simulink model "PILnewH2019"  (R2021a)
settings: Solver=FixedStepAuto  StartTime=0.0  StopTime=41.24  FixedStep=0.001  RelTol=1e-3  EnableMultiTasking=on
values from neighbouring files (symbols this model uses):
  den_lpf_d = den_lpf20    [Mainframe_init.m]    (also in load_autopilot.m)
  Emulated_FCC_IO_Delay = 7    [Mainframe_init.m]
  Enable_Gyros = 0    [Mainframe_init.m]
  Enable_INS = 0    [Mainframe_init.m]
  num_lpf_d = num_lpf20    [Mainframe_init.m]    (also in load_autopilot.m)
undefined symbols (not defined in the file or in its folder): act_dmp, act_omega, Actuator, Aerodynamics, aMode, Autopilot, AUX, c_b_WGS, c_be, c_flat, c_grav, c_h_geop0, c_h_geope, c_pa0, c_pe, c_r0, c_rot, c_rsma, c_Tmp0, d_siB_0, d_siB_max, d_siB_min, dd_siB_max, dd_siB_min, dev, DiscIntNeverNeededParam, e_pa, e_Tmp, Earth, fin_maxrate, flag_I_act_switch, flag_I_aero_switch, flag_I_flat, flag_I_gravity_switch, flag_I_rot, hcr, HIL_Data, JMMM_0, JMMM_e, JSPB_e, lat_0, lon_0, Mass_Props, mB_0, mM_0, mM_e, National_Instruments, pBII_0, PCIe, pMPB, pNPB, propellant_kg, prp_FBPB, prp_mdot, prp_T, pSPB, pwm_output1, qEG_0, qIB_0, qIE_0 ... (+29)
libraries: simulink x31, simulink_extras x24, aerolibcommonsys x4, px4lib x2, custom_blocks x1, pil_lib x1, aerolibtransform2 x1, sldrtlib x1, aerolibnav x1
(part 10 of 15)

== system PILnewH2019/Non-linear Flight Dynamic Model/Subsystem1/GRM_Airframe/stream_flow/calc_stream_flow/velocity_vector_transformation ==
  wIEE : Inport
  TIE : Inport  Port=2
  vBII : Inport  Port=3
  pBII : Inport  Port=4
  Add : Sum  Inputs=+-
  Product : Product  Multiplication=Matrix(*)
  cross_product : Subsystem
      mask help: cross product r3 = r1 x r2
      mask Help:
      | Name:
      | 
      |     cross_product
      | 
      | Description:
      | 
      |     This block implements the cross product r3 = r1 x r2.
      | 
      | Inputs  [size] [data type] [unit]:
      | 
      |     vector 1  [3] [double] [-]
      |     vector 2  [3] [double] [-]
      | 
      | Outputs  [size] [data type] [unit]:
      | 
      |     resulting vector  [3] [double] [-]
      mask Display: disp(' r3 = r1 x r2')
  vBEI : Outport  VectorParamsAs1DForOutWhenUnconnected=off
  wires:
  TIE/1 -> Product/1
  wIEE/1 -> Product/2
  Product/1 -> cross_product/1(r1)  "wIEI"
  pBII/1 -> cross_product/2(r2)
  cross_product/1(r1_x_r2) -> Add/2  "de_vBEI"
  vBII/1 -> Add/1
  Add/1 -> vBEI/1  "vBEI"

== system PILnewH2019/Non-linear Flight Dynamic Model/Subsystem1/GRM_Airframe/weight_and_balance/moi/JMMM_linear_interpolation ==
  mM : Inport
  Constant16 : Constant  Value=JMMM_0
  Constant17 : Constant  Value=JMMM_e
  Constant18 : Constant  Value=mM_0
  Constant19 : Constant  Value=mM_e
  Constant20 : Constant  Value=mM_0
  Constant21 : Constant  Value=JMMM_0
  Divide : Product  Inputs=**/
  Subtract : Sum  Inputs=+-
  Subtract4 : Sum  Inputs=+-
  Subtract5 : Sum  Inputs=+-
  Subtract6 : Sum
  JMMM : Outport  VectorParamsAs1DForOutWhenUnconnected=off
  wires:
  mM/1 -> Subtract5/1
  Subtract5/1 -> Divide/1
  Constant20/1 -> Subtract5/2
  Constant19/1 -> Subtract4/1
  Constant18/1 -> Subtract4/2
  Constant17/1 -> Subtract/1
  Constant16/1 -> Subtract/2
  Subtract/1 -> Divide/2
  Subtract4/1 -> Divide/3
  Subtract6/1 -> JMMM/1  "JMMM"
  Constant21/1 -> Subtract6/1
  Divide/1 -> Subtract6/2

== system PILnewH2019/Non-linear Flight Dynamic Model/Subsystem1/GRM_Airframe/weight_and_balance/moi/moi_coordinate_transformation ==
  JMMM : Inport
  3_rot_mat : Subsystem  mask(Rotation um 1, 2 oder 3 Achsen){rot_1=Rotation um z-Achse, rot_2=Rotation um y-Achse, rot_3=Rotation um x-Achse}
      mask prompts: rot_1 "1. Rotation"; rot_2 "2. Rotation"; rot_3 "3. Rotation"
      mask help:
      | Dieser Block liefert die Rotationsmatrix T12 für den Fall zurück, dass sich das Ziel-Koordinatensystem (1) durch Drehungen um 1, 2 oder 3 Achsen gegenüber dem Ausgangskoordinatensystem (2) beschreiben lässt (passive Drehung).
      |
      | Die Anzahl der Rotation sowie die Reihenfolge ist frei einstellbar.
      |
      | Die Rotationswinkel haben die Einheit [rad].
      mask TypeOptions rot_1: Rotation um x-Achse | Rotation um y-Achse | Rotation um z-Achse
      mask TypeOptions rot_2: Rotation um x-Achse | Rotation um y-Achse | Rotation um z-Achse
      mask TypeOptions rot_3: Rotation um x-Achse | Rotation um y-Achse | Rotation um z-Achse
  Math Function : Math  Operator=transpose  SignedPower=on  SaturateOnIntegerOverflow=on
  Matrix Multiply : Product  Multiplication=Matrix(*)
  Matrix Multiply1 : Product  Multiplication=Matrix(*)
  Thrust_rot_z : Constant  Value=unc_prp_z
  thrust_rot_x : Constant  Value=unc_prp_x
  thrust_rot_y : Constant  Value=unc_prp_y
  JMMB : Outport  VectorParamsAs1DForOutWhenUnconnected=off
  wires:
  Math Function/1 -> Matrix Multiply1/2
  Matrix Multiply/1 -> Matrix Multiply1/1
  JMMM/1 -> Matrix Multiply/2
  3_rot_mat/1(T12) -> Math Function/1, Matrix Multiply/1
  Matrix Multiply1/1 -> JMMB/1  "JMMB"
  thrust_rot_y/1 -> 3_rot_mat/2(wi2)
  thrust_rot_x/1 -> 3_rot_mat/3(wi3)
  Thrust_rot_z/1 -> 3_rot_mat/1(wi1)

== system PILnewH2019/Non-linear Flight Dynamic Model/Subsystem1/GRM_Airframe/weight_and_balance/moi/moi_uncertainty ==
  JBBB_c : Inport
  Add7 : Sum
  Constant16 : Constant  Value=[unc_moi_Jxx,0,0;0,unc_moi_Jyy,0;0,0,unc_moi_Jzz]
  JBBB : Outport  VectorParamsAs1DForOutWhenUnconnected=off
  wires:
  Add7/1 -> JBBB/1  "JBBB"
  JBBB_c/1 -> Add7/1
  Constant16/1 -> Add7/2

== system PILnewH2019/Non-linear Flight Dynamic Model/Subsystem1/GRM_Airframe/weight_and_balance/moi/steiners_theorem_missile ==
  pBPB : Inport
  Constant : Constant  Value=mB_0
  Constant17 : Constant  Value=pSPB
  Product : Product
  Subtract : Sum  Inputs=+-
  create_deviation_matrix : Subsystem
  J_deviation : Outport  VectorParamsAs1DForOutWhenUnconnected=off
  wires:
  pBPB/1 -> Subtract/1
  Product/1 -> J_deviation/1
  create_deviation_matrix/1(T_deviation) -> Product/2
  Constant17/1 -> Subtract/2
  Subtract/1 -> create_deviation_matrix/1(pBXB)  "pB0B"
  Constant/1 -> Product/1

== system PILnewH2019/Non-linear Flight Dynamic Model/Subsystem1/GRM_Airframe/weight_and_balance/moi/steiners_theorem_motor ==
  pBPB : Inport
  mM : Inport  Port=2
  Constant16 : Constant  Value=pMPB
  Product : Product
  Subtract4 : Sum  Inputs=+-
  create_deviation_matrix1 : Subsystem
  JM_deviation : Outport  VectorParamsAs1DForOutWhenUnconnected=off
  wires:
  Product/1 -> JM_deviation/1
  pBPB/1 -> Subtract4/1
  create_deviation_matrix1/1(T_deviation) -> Product/1
  Constant16/1 -> Subtract4/2
  Subtract4/1 -> create_deviation_matrix1/1(pBXB)  "pBMB"
  mM/1 -> Product/2

== system PILnewH2019/Flight Control Computer/FCC - Real or Emulated/Emulated FCC/PixBlock3/Emulated Pixhawk/Autopilot/Calculate U ==
  INS Data : Inport
  Add : Sum  Inputs=+++
  Bus Selector1 : BusSelector  OutputSignals=u,v,w
  Square : Math  Operator=square  SaturateOnIntegerOverflow=on
  Square Root : Sqrt  SaturateOnIntegerOverflow=on
  Square1 : Math  Operator=square  SaturateOnIntegerOverflow=on
  Square2 : Math  Operator=square  SaturateOnIntegerOverflow=on
  U : Outport
  wires:
  Square/1 -> Add/1
  Square2/1 -> Add/3
  Square Root/1 -> U/1
  Add/1 -> Square Root/1
  Square1/1 -> Add/2
  Bus Selector1/2 -> Square1/1  "<v>"
  Bus Selector1/3 -> Square2/1  "<w>"
  Bus Selector1/1 -> Square/1  "<u>"
  INS Data/1 -> Bus Selector1/1

== system PILnewH2019/Flight Control Computer/FCC - Real or Emulated/Emulated FCC/PixBlock3/Emulated Pixhawk/Autopilot/Phi_Control ==
  phi_cmd_rad : Inport
  phi_rad : Inport  Port=2
  p_rps : Inport  Port=3
  Reset Integrators : Inport  Port=4
  V_mps : Inport  Port=5
  h_m : Inport  Port=6
  Bus Selector : BusSelector  OutputSignals=Kp_p,Ki_phi,Kp_phi,Kp_r,Ki_ay,Kp_ay
  Constant : Constant  Value=0  OutDataTypeStr=single
  Discrete-Time Integrator : DiscreteIntegrator  ExternalReset=level  InitialConditionSource=external  SampleTime=-1  OutDataTypeStr=single  ICPrevOutput=DiscIntNeverNeededParam  ICPrevScaledInput=DiscIntNeverNeededParam
  Gain_Lookup : Subsystem
  Product1 : Product
  Product2 : Product
  Product3 : Product
  Sum3 : Sum  Inputs=|+-
  Sum4 : Sum  Inputs=++|
  Sum5 : Sum  Inputs=|+-
  dela_cmd_rad : Outport
  wires:
  phi_cmd_rad/1 -> Sum3/1
  Reset Integrators/1 -> Discrete-Time Integrator/2
  p_rps/1 -> Sum5/2
  phi_rad/1 -> Sum3/2
  Product2/1 -> Sum4/1
  Sum3/1 -> Product3/2, Product2/2
  Constant/1 -> Discrete-Time Integrator/3
  Sum5/1 -> Product1/2
  [Ki_phi] -> Product3/1
  Product1/1 -> dela_cmd_rad/1
  [Kp_p] -> Product1/1
  [Kp_phi] -> Product2/1
  Discrete-Time Integrator/1 -> Sum4/2  "phi_int"
  Sum4/1 -> Sum5/1
  Product3/1 -> Discrete-Time Integrator/1
  h_m/1 -> Gain_Lookup/2(h_m)
  Bus Selector/6 -> [Kp_ay]  "<Kp_ay>"
  Bus Selector/5 -> [Ki_ay]  "<Ki_ay>"
  Bus Selector/2 -> [Ki_phi]  "<Ki_phi>"
  Bus Selector/1 -> [Kp_p]  "<Kp_p>"
  V_mps/1 -> Gain_Lookup/1(V_mps)
  Bus Selector/4 -> [Kp_r]  "<Kp_r>"
  Gain_Lookup/1(Gains) -> Bus Selector/1
  Bus Selector/3 -> [Kp_phi]  "<Kp_phi>"

== system PILnewH2019/Flight Control Computer/FCC - Real or Emulated/Emulated FCC/PixBlock3/Emulated Pixhawk/Convert to Bus/100Hz Reset ==
  Heartbeat : Inport
  Delay : Delay  DelayLength=1
  GreaterThan : RelationalOperator  Operator=<  OutDataTypeStr=boolean  RndMeth=Simplest
  RST : Outport
  wires:
  GreaterThan/1 -> RST/1
  Delay/1 -> GreaterThan/2
  Heartbeat/1 -> Delay/1, GreaterThan/1

== system PILnewH2019/Flight Control Computer/FCC - Real or Emulated/Emulated FCC/PixBlock3/Emulated Pixhawk/Fin Allocation/control_allocation ==
  fin_cmd : Inport
  Constant7 : Constant  Value=HIL_Data.FDM.Tr4r3  OutDataTypeStr=single
  Product : Product  Multiplication=Matrix(*)
  siB_cmd : Outport  VectorParamsAs1DForOutWhenUnconnected=off
  wires:
  Constant7/1 -> Product/1
  fin_cmd/1 -> Product/2
  Product/1 -> siB_cmd/1  "siB_cmd"

== system PILnewH2019/Flight Control Computer/FCC - Real or Emulated/Emulated FCC/PixBlock3/Emulated Pixhawk/Inertial Navigation System/INS (INCOMPLETE) ==
  IMU Data : Inport
  Bus Creator2 : BusCreator  Inputs=12
  One{,1..11} (12 alike) : Constant  Value=-1  OutDataTypeStr=Inherit: Inherit via back propagation
  Terminator : Terminator
  INS Data : Outport
  wires:
  One11/1 -> Bus Creator2/12  "psi"
  One10/1 -> Bus Creator2/11  "theta"
  One9/1 -> Bus Creator2/10  "phi"
  One8/1 -> Bus Creator2/9  "r"
  One7/1 -> Bus Creator2/8  "q"
  One2/1 -> Bus Creator2/3  "w"
  One6/1 -> Bus Creator2/7  "p"
  One4/1 -> Bus Creator2/5  "y"
  One1/1 -> Bus Creator2/2  "v"
  One5/1 -> Bus Creator2/6  "z"
  One/1 -> Bus Creator2/1  "u"
  One3/1 -> Bus Creator2/4  "x"
  IMU Data/1 -> Terminator/1
  Bus Creator2/1 -> INS Data/1

== system PILnewH2019/Flight Control Computer/FCC - Real or Emulated/Emulated FCC/PixBlock3/Emulated Pixhawk/Servo Commands/100Hz Progress ==
  Delay : Delay  DelayLength=1
  GreaterThan : RelationalOperator  Operator=>  OutDataTypeStr=boolean  RndMeth=Simplest
  RST : Outport
  wires:
  GreaterThan/1 -> RST/1
  Delay/1 -> GreaterThan/2
  [Heartbeat] -> Delay/1, GreaterThan/1

== system PILnewH2019/Flight Control Computer/FCC - Real or Emulated/Real FCC/PixBlock2/Emulated Pixhawk/Autopilot/Calculate U ==
  INS Data : Inport
  Add : Sum  Inputs=+++
  Bus Selector1 : BusSelector  OutputSignals=u,v,w
  Square : Math  Operator=square  SaturateOnIntegerOverflow=on
  Square Root : Sqrt  SaturateOnIntegerOverflow=on
  Square1 : Math  Operator=square  SaturateOnIntegerOverflow=on
  Square2 : Math  Operator=square  SaturateOnIntegerOverflow=on
  U : Outport
  wires:
  Square/1 -> Add/1
  Square2/1 -> Add/3
  Square Root/1 -> U/1
  Add/1 -> Square Root/1
  Square1/1 -> Add/2
  Bus Selector1/2 -> Square1/1  "<v>"
  Bus Selector1/3 -> Square2/1  "<w>"
  Bus Selector1/1 -> Square/1  "<u>"
  INS Data/1 -> Bus Selector1/1

== system PILnewH2019/Flight Control Computer/FCC - Real or Emulated/Real FCC/PixBlock2/Emulated Pixhawk/Autopilot/Phi_Control ==
  phi_cmd_rad : Inport
  phi_rad : Inport  Port=2
  p_rps : Inport  Port=3
  Reset Integrators : Inport  Port=4
  V_mps : Inport  Port=5
  h_m : Inport  Port=6
  Bus Selector : BusSelector  OutputSignals=Kp_p,Ki_phi,Kp_phi,Kp_r,Ki_ay,Kp_ay
  Constant : Constant  Value=0  OutDataTypeStr=single
  Discrete-Time Integrator : DiscreteIntegrator  ExternalReset=level  InitialConditionSource=external  SampleTime=-1  OutDataTypeStr=single  ICPrevOutput=DiscIntNeverNeededParam  ICPrevScaledInput=DiscIntNeverNeededParam
  Gain_Lookup : Subsystem
  Product1 : Product
  Product2 : Product
  Product3 : Product
  Sum3 : Sum  Inputs=|+-
  Sum4 : Sum  Inputs=++|
  Sum5 : Sum  Inputs=|+-
  dela_cmd_rad : Outport
  wires:
  phi_cmd_rad/1 -> Sum3/1
  Reset Integrators/1 -> Discrete-Time Integrator/2
  p_rps/1 -> Sum5/2
  phi_rad/1 -> Sum3/2
  Product2/1 -> Sum4/1
  Sum3/1 -> Product3/2, Product2/2
  Constant/1 -> Discrete-Time Integrator/3
  Sum5/1 -> Product1/2
  [Ki_phi] -> Product3/1
  Product1/1 -> dela_cmd_rad/1
  [Kp_p] -> Product1/1
  [Kp_phi] -> Product2/1
  Discrete-Time Integrator/1 -> Sum4/2  "phi_int"
  Sum4/1 -> Sum5/1
  Product3/1 -> Discrete-Time Integrator/1
  h_m/1 -> Gain_Lookup/2(h_m)
  Bus Selector/6 -> [Kp_ay]  "<Kp_ay>"
  Bus Selector/5 -> [Ki_ay]  "<Ki_ay>"
  Bus Selector/2 -> [Ki_phi]  "<Ki_phi>"
  Bus Selector/1 -> [Kp_p]  "<Kp_p>"
  V_mps/1 -> Gain_Lookup/1(V_mps)
  Bus Selector/4 -> [Kp_r]  "<Kp_r>"
  Gain_Lookup/1(Gains) -> Bus Selector/1
  Bus Selector/3 -> [Kp_phi]  "<Kp_phi>"

== system PILnewH2019/Flight Control Computer/FCC - Real or Emulated/Real FCC/PixBlock2/Emulated Pixhawk/Convert to Bus/100Hz Reset ==
  Heartbeat : Inport
  Delay : Delay  DelayLength=1
  GreaterThan : RelationalOperator  Operator=<  OutDataTypeStr=boolean  RndMeth=Simplest
  RST : Outport
  wires:
  GreaterThan/1 -> RST/1
  Delay/1 -> GreaterThan/2
  Heartbeat/1 -> Delay/1, GreaterThan/1

== system PILnewH2019/Flight Control Computer/FCC - Real or Emulated/Real FCC/PixBlock2/Emulated Pixhawk/Fin Allocation/control_allocation ==
  fin_cmd : Inport
  Constant7 : Constant  Value=HIL_Data.FDM.Tr4r3  OutDataTypeStr=single
  Product : Product  Multiplication=Matrix(*)
  siB_cmd : Outport  VectorParamsAs1DForOutWhenUnconnected=off
  wires:
  Constant7/1 -> Product/1
  fin_cmd/1 -> Product/2
  Product/1 -> siB_cmd/1  "siB_cmd"

== system PILnewH2019/Flight Control Computer/FCC - Real or Emulated/Real FCC/PixBlock2/Emulated Pixhawk/Inertial Navigation System/INS (INCOMPLETE) ==
  IMU Data : Inport
  Bus Creator2 : BusCreator  Inputs=12
  One{,1..11} (12 alike) : Constant  Value=-1  OutDataTypeStr=Inherit: Inherit via back propagation
  Terminator : Terminator
  INS Data : Outport
  wires:
  One11/1 -> Bus Creator2/12  "psi"
  One10/1 -> Bus Creator2/11  "theta"
  One9/1 -> Bus Creator2/10  "phi"
  One8/1 -> Bus Creator2/9  "r"
  One7/1 -> Bus Creator2/8  "q"
  One2/1 -> Bus Creator2/3  "w"
  One6/1 -> Bus Creator2/7  "p"
  One4/1 -> Bus Creator2/5  "y"
  One1/1 -> Bus Creator2/2  "v"
  One5/1 -> Bus Creator2/6  "z"
  One/1 -> Bus Creator2/1  "u"
  One3/1 -> Bus Creator2/4  "x"
  IMU Data/1 -> Terminator/1
  Bus Creator2/1 -> INS Data/1

== system PILnewH2019/Flight Control Computer/FCC - Real or Emulated/Real FCC/PixBlock2/Emulated Pixhawk/Servo Commands/100Hz Progress ==
  Delay : Delay  DelayLength=1
  GreaterThan : RelationalOperator  Operator=>  OutDataTypeStr=boolean  RndMeth=Simplest
  RST : Outport
  wires:
  GreaterThan/1 -> RST/1
  Delay/1 -> GreaterThan/2
  [Heartbeat] -> Delay/1, GreaterThan/1

== system PILnewH2019/Non-linear Flight Dynamic Model/Extract States/Assemble_States_Bus1/Three-axis Inertial Measurement Unit3/Three-axis Accelerometer/Dynamics/No Dynamics ==
  In1 : Inport
  Out1 : Outport  VectorParamsAs1DForOutWhenUnconnected=off
  wires:
  In1/1 -> Out1/1

== system PILnewH2019/Non-linear Flight Dynamic Model/Extract States/Assemble_States_Bus1/Three-axis Inertial Measurement Unit3/Three-axis Accelerometer/Dynamics/Second-order Dynamics ==
  In : Inport
  2*zeta * wn : Gain  Gain=2.0*zn*wn  SaturateOnIntegerOverflow=on  OutDataTypeStr=Inherit: Same as input  ParamDataTypeStr=Inherit: Same as input
  "Integrator, Second-Order Limited" : SecondOrderIntegrator  ICX=0  UpperLimitX=fin_max  LowerLimitX=fin_min  ICDXDT=0  UpperLimitDXDT=fin_maxrate  LowerLimitDXDT=-fin_maxrate
  Sum2 : Sum  Inputs=|+-  InputSameDT=on  SaturateOnIntegerOverflow=on  OutDataTypeStr=Inherit: Same as first input
  Sum3 : Sum  Inputs=|+-  InputSameDT=on  SaturateOnIntegerOverflow=on  OutDataTypeStr=Inherit: Same as first input
  wn^2 : Gain  Gain=wn*wn  SaturateOnIntegerOverflow=on  OutDataTypeStr=Inherit: Same as input  ParamDataTypeStr=Inherit: Same as input
  Out : Outport  VectorParamsAs1DForOutWhenUnconnected=off
  wires:
  "Integrator, Second-Order Limited"/2 -> 2*zeta * wn/1
  "Integrator, Second-Order Limited"/1 -> Out/1, Sum3/2
  wn^2/1 -> Sum2/1
  Sum3/1 -> wn^2/1
  2*zeta * wn/1 -> Sum2/2
  Sum2/1 -> "Integrator, Second-Order Limited"/1
  In/1 -> Sum3/1

== system PILnewH2019/Non-linear Flight Dynamic Model/Extract States/Assemble_States_Bus1/Three-axis Inertial Measurement Unit3/Three-axis Accelerometer/w x (w x d)/w x (w x d) ==
  A : Inport
  B : Inport  Port=2
  "A " : InportShadow
  "B " : InportShadow  Port=2
  Subsystem : Subsystem
  Subsystem1 : Subsystem
  Sum : Sum  Inputs=+|-  InputSameDT=on  SaturateOnIntegerOverflow=on  OutDataTypeStr=Inherit: Same as first input
  C : Outport  VectorParamsAs1DForOutWhenUnconnected=off
  wires:
  Subsystem1/1(Out1) -> Sum/2
  Subsystem/1(Out1) -> Sum/1
  A/1 -> Subsystem/1(A)
  B/1 -> Subsystem/2(B)
  Sum/1 -> C/1
  "A "/1 -> Subsystem1/1(A)
  "B "/1 -> Subsystem1/2(B)

== system PILnewH2019/Non-linear Flight Dynamic Model/Extract States/Assemble_States_Bus1/Three-axis Inertial Measurement Unit3/Three-axis Accelerometer/w x (w x d)/w x d ==
  A : Inport
  B : Inport  Port=2
  "A " : InportShadow
  "B " : InportShadow  Port=2
  Subsystem : Subsystem
  Subsystem1 : Subsystem
  Sum : Sum  Inputs=+|-  InputSameDT=on  SaturateOnIntegerOverflow=on  OutDataTypeStr=Inherit: Same as first input
  C : Outport  VectorParamsAs1DForOutWhenUnconnected=off
  wires:
  Subsystem1/1(Out1) -> Sum/2
  Subsystem/1(Out1) -> Sum/1
  A/1 -> Subsystem/1(A)
  B/1 -> Subsystem/2(B)
  Sum/1 -> C/1
  "A "/1 -> Subsystem1/1(A)
  "B "/1 -> Subsystem1/2(B)

== system PILnewH2019/Non-linear Flight Dynamic Model/Extract States/Assemble_States_Bus1/Three-axis Inertial Measurement Unit3/Three-axis Accelerometer/wdot x d/Subsystem ==
  A : Inport
  B : Inport  Port=2
  Demux : Demux  Outputs=3
  Demux1 : Demux  Outputs=3
  Mux : Mux  Inputs=3
  i x j : Product  InputSameDT=on  SaturateOnIntegerOverflow=on  OutDataTypeStr=Inherit: Same as first input
  j x k : Product  InputSameDT=on  SaturateOnIntegerOverflow=on  OutDataTypeStr=Inherit: Same as first input
  k x i : Product  InputSameDT=on  SaturateOnIntegerOverflow=on  OutDataTypeStr=Inherit: Same as first input
  Out1 : Outport  VectorParamsAs1DForOutWhenUnconnected=off
  wires:
  Mux/1 -> Out1/1
  A/1 -> Demux/1
  B/1 -> Demux1/1
  j x k/1 -> Mux/1
  k x i/1 -> Mux/2
  i x j/1 -> Mux/3
  Demux/1 -> i x j/1
  Demux1/2 -> i x j/2
  Demux1/1 -> k x i/2
  Demux/3 -> k x i/1
  Demux/2 -> j x k/1
  Demux1/3 -> j x k/2

== system PILnewH2019/Non-linear Flight Dynamic Model/Extract States/Assemble_States_Bus1/Three-axis Inertial Measurement Unit3/Three-axis Accelerometer/wdot x d/Subsystem1 ==
  A : Inport
  B : Inport  Port=2
  Demux : Demux  Outputs=3
  Demux1 : Demux  Outputs=3
  Mux : Mux  Inputs=3
  i x k : Product  InputSameDT=on  SaturateOnIntegerOverflow=on  OutDataTypeStr=Inherit: Same as first input
  j x i : Product  InputSameDT=on  SaturateOnIntegerOverflow=on  OutDataTypeStr=Inherit: Same as first input
  k x j : Product  InputSameDT=on  SaturateOnIntegerOverflow=on  OutDataTypeStr=Inherit: Same as first input
  Out1 : Outport  VectorParamsAs1DForOutWhenUnconnected=off
  wires:
  A/1 -> Demux/1
  B/1 -> Demux1/1
  Demux/3 -> k x j/1
  Demux1/2 -> k x j/2
  Demux/1 -> i x k/1
  Demux1/3 -> i x k/2
  Demux/2 -> j x i/1
  Demux1/1 -> j x i/2
  Mux/1 -> Out1/1
  k x j/1 -> Mux/1
  i x k/1 -> Mux/2
  j x i/1 -> Mux/3

== system PILnewH2019/Non-linear Flight Dynamic Model/Extract States/Assemble_States_Bus1/Three-axis Inertial Measurement Unit3/Three-axis Gyroscope/Dynamics/No Dynamics ==
  In1 : Inport
  Out1 : Outport  VectorParamsAs1DForOutWhenUnconnected=off
  wires:
  In1/1 -> Out1/1

== system PILnewH2019/Non-linear Flight Dynamic Model/Extract States/Assemble_States_Bus1/Three-axis Inertial Measurement Unit3/Three-axis Gyroscope/Dynamics/Second-order Dynamics ==
  In : Inport
  2*zeta * wn : Gain  Gain=2.0*zn*wn  SaturateOnIntegerOverflow=on  OutDataTypeStr=Inherit: Same as input  ParamDataTypeStr=Inherit: Same as input
  "Integrator, Second-Order Limited" : SecondOrderIntegrator  ICX=0  UpperLimitX=fin_max  LowerLimitX=fin_min  ICDXDT=0  UpperLimitDXDT=fin_maxrate  LowerLimitDXDT=-fin_maxrate
  Sum2 : Sum  Inputs=|+-  InputSameDT=on  SaturateOnIntegerOverflow=on  OutDataTypeStr=Inherit: Same as first input
  Sum3 : Sum  Inputs=|+-  InputSameDT=on  SaturateOnIntegerOverflow=on  OutDataTypeStr=Inherit: Same as first input
  wn^2 : Gain  Gain=wn*wn  SaturateOnIntegerOverflow=on  OutDataTypeStr=Inherit: Same as input  ParamDataTypeStr=Inherit: Same as input
  Out : Outport  VectorParamsAs1DForOutWhenUnconnected=off
  wires:
  "Integrator, Second-Order Limited"/2 -> 2*zeta * wn/1
  "Integrator, Second-Order Limited"/1 -> Out/1, Sum3/2
  wn^2/1 -> Sum2/1
  Sum3/1 -> wn^2/1
  2*zeta * wn/1 -> Sum2/2
  Sum2/1 -> "Integrator, Second-Order Limited"/1
  In/1 -> Sum3/1

== system PILnewH2019/Non-linear Flight Dynamic Model/GRM_Airframe/aerodynamics/aerodynamic_via_lookup/calc_aero_for_mom/launch_rail/initial_altitude ==
  Constant : Constant  Value=pBII_0
  Constant2 : Constant  Value=flag_I_flat
  Demux : Demux  Outputs=3
  Gain : Gain  Gain=-1
  Switch1 : Switch  Criteria=u2 > Threshold
  Terminator{,1..3} (4 alike) : Terminator
  trafo_E_to_geodetic : Subsystem  mask(Transformation der ECEF Position in geodätische Größen){}
      mask help: Dieser Block transformiert die Position im ECEF KOS in die geodätische Länge, Breite und Höhe
      mask init:
      | [c_mue, c_rsma, c_flat] = init_transformations_earth;
      mask Help:
      | Name:
      | 
      |     trafo_E_to_geodetic
      | 
      | Beschreibung:
      | 
      |     Dieser Block transformiert die Position im ECEF KOS in die geodätische
      |     Länge, Breite und Höhe.
      | 
      | Inputs   [size]  [data type] [unit]:
      | 
      |     pBEE    [3] [double] [m]
      | 
      | Outputs  [size]  [data type] [unit]:
      | 
      |     long  [1] [double] [rad]
      |     lat   [1] [double] [rad]
      |     alt   [1] [double] [m]
      | 
      | Parameter
      | 
      |    c_rsma
      |    c_flat
  hBE_0 : Outport  VectorParamsAs1DForOutWhenUnconnected=off
  wires:
  Constant2/1 -> Switch1/2
  trafo_E_to_geodetic/3(alt) -> Switch1/3  "hBE_0"
  Demux/2 -> Terminator3/1
  Demux/3 -> Gain/1
  Gain/1 -> Switch1/1
  Demux/1 -> Terminator2/1
  trafo_E_to_geodetic/2(lat) -> Terminator1/1
  Constant/1 -> Demux/1, trafo_E_to_geodetic/1(pBEE)
  trafo_E_to_geodetic/1(lon) -> Terminator/1
  Switch1/1 -> hBE_0/1  "hBE_0"

== system PILnewH2019/Non-linear Flight Dynamic Model/GRM_Airframe/aerodynamics/aerodynamic_via_lookup/calc_aero_for_mom/launch_rail1/initial_altitude ==
  Constant : Constant  Value=pBII_0
  Constant2 : Constant  Value=flag_I_flat
  Demux : Demux  Outputs=3
  Gain : Gain  Gain=-1
  Switch1 : Switch  Criteria=u2 > Threshold
  Terminator{,1..3} (4 alike) : Terminator
  trafo_E_to_geodetic : Subsystem  mask(Transformation der ECEF Position in geodätische Größen){}
      mask help: Dieser Block transformiert die Position im ECEF KOS in die geodätische Länge, Breite und Höhe
      mask init:
      | [c_mue, c_rsma, c_flat] = init_transformations_earth;
      mask Help:
      | Name:
      | 
      |     trafo_E_to_geodetic
      | 
      | Beschreibung:
      | 
      |     Dieser Block transformiert die Position im ECEF KOS in die geodätische
      |     Länge, Breite und Höhe.
      | 
      | Inputs   [size]  [data type] [unit]:
      | 
      |     pBEE    [3] [double] [m]
      | 
      | Outputs  [size]  [data type] [unit]:
      | 
      |     long  [1] [double] [rad]
      |     lat   [1] [double] [rad]
      |     alt   [1] [double] [m]
      | 
      | Parameter
      | 
      |    c_rsma
      |    c_flat
  hBE_0 : Outport  VectorParamsAs1DForOutWhenUnconnected=off
  wires:
  Switch1/1 -> hBE_0/1  "hBE_0"
  trafo_E_to_geodetic/1(lon) -> Terminator/1
  Constant/1 -> trafo_E_to_geodetic/1(pBEE), Demux/1
  trafo_E_to_geodetic/2(lat) -> Terminator1/1
  Demux/1 -> Terminator2/1
  Gain/1 -> Switch1/1
  Demux/3 -> Gain/1
  Demux/2 -> Terminator3/1
  trafo_E_to_geodetic/3(alt) -> Switch1/3  "hBE_0"
  Constant2/1 -> Switch1/2

== system PILnewH2019/Non-linear Flight Dynamic Model/GRM_Airframe/environment/WGS84_Gravitation/WGS84_2_ECEF/WGS84 Transformation Parameter /Subsystem ==
  b : Inport
  a : Inport  Port=2
  Add : Sum  Inputs=-+
  Add1 : Sum  Inputs=+-
  Divide : Product  Inputs=*/
  Divide1 : Product  Inputs=**
  Sqrt : Sqrt  SaturateOnIntegerOverflow=on
  a2 : Constant  Value=2
  e : Outport  VectorParamsAs1DForOutWhenUnconnected=off
  wires:
  Sqrt/1 -> e/1  "e"
  a/1 -> Add/2, Divide/2
  b/1 -> Add/1
  a2/1 -> Add1/1
  Divide1/1 -> Sqrt/1
  Divide/1 -> Divide1/2, Add1/2  "f"
  Add1/1 -> Divide1/1
  Add/1 -> Divide/1

== system PILnewH2019/Non-linear Flight Dynamic Model/GRM_Airframe/gravity/launch_rail/initial_altitude/trafo_E_to_geodetic/Geodetic_altitude ==
  pBEE : Inport
  c_rsma : Inport  Port=2
  c_flat : Inport  Port=3
  lat : Inport  Port=4
  Add : Sum
  Constant : Constant
  Gain : Gain  Gain=2
  Product : Product  Inputs=*/  InputSameDT=on  RndMeth=Zero  SaturateOnIntegerOverflow=on  OutDataTypeStr=Inherit: Same as first input
  Product1 : Product
  Product2 : Product
  Product3 : Product
  Product4 : Product  Inputs=*/  InputSameDT=on  RndMeth=Zero  SaturateOnIntegerOverflow=on  OutDataTypeStr=Inherit: Same as first input
  Product5 : Product  Inputs=3
  Selector : Selector  IndexMode=Zero-based  InputPortWidth=3  IndexOptions=Index vector (dialog)  Indices=0  OutputSizes=1
  Selector1 : Selector  IndexMode=Zero-based  InputPortWidth=3  IndexOptions=Index vector (dialog)  Indices=1  OutputSizes=1
  Sqrt : Sqrt  SaturateOnIntegerOverflow=on
  Sqrt1 : Sqrt  SaturateOnIntegerOverflow=on
  Subtract : Sum  Inputs=+-
  Subtract1 : Sum  Inputs=+-
  Sum : Sum  Inputs=+-  InputSameDT=on  SaturateOnIntegerOverflow=on  OutDataTypeStr=Inherit: Same as first input
  Trigonometric Function : Trigonometry
  cos(latGD) : Trigonometry  Operator=cos
  alt : Outport  VectorParamsAs1DForOutWhenUnconnected=off
  wires:
  Product4/1 -> Sum/2
  Trigonometric Function/1 -> Product5/1, Product5/2
  Product5/1 -> Subtract1/2
  Constant/1 -> Subtract1/1
  Subtract1/1 -> Sqrt1/1
  Sqrt1/1 -> Product4/2
  c_flat/1 -> Gain/1, Product3/2, Product3/1
  Gain/1 -> Subtract/1
  Product3/1 -> Subtract/2
  pBEE/1 -> Selector/1, Selector1/1
  Add/1 -> Sqrt/1
  Product2/1 -> Add/2
  Product1/1 -> Add/1
  Selector1/1 -> Product2/1, Product2/2
  Selector/1 -> Product1/1, Product1/2
  Sum/1 -> alt/1  "alt"
  Product/1 -> Sum/1
  Subtract/1 -> Product5/3
  c_rsma/1 -> Product4/1
  cos(latGD)/1 -> Product/2
  Sqrt/1 -> Product/1
  lat/1 -> cos(latGD)/1, Trigonometric Function/1

== system PILnewH2019/Non-linear Flight Dynamic Model/GRM_Airframe/gravity/launch_rail/initial_altitude/trafo_E_to_geodetic/Geodetic_latitude ==
  pBEE : Inport
  c_rsma : Inport  Port=2
  c_flat : Inport  Port=3
  Add : Sum
  Add1 : Sum
  Constant : Constant
  Demux1 : Demux  Outputs=[1;1;1]
      settings: DisplayOption=none
  Divide : Product  Inputs=*/
  Divide1 : Product  Inputs=*/
  Divide2 : Product  Inputs=*/
  Gain : Gain  Gain=2
  Product{,1..7} (8 alike) : Product
  Product{8..11} (4 alike) : Product  Inputs=3
  Sqrt : Sqrt  SaturateOnIntegerOverflow=on
  Subtract{,1..3} (4 alike) : Sum  Inputs=+-
  Trigonometric Function : Trigonometry  Operator=atan
  Trigonometric Function1 : Trigonometry  Operator=atan
  Trigonometric Function2 : Trigonometry
  Trigonometric Function3 : Trigonometry  Operator=cos
  lat : Outport  VectorParamsAs1DForOutWhenUnconnected=off
  wires:
  Divide/1 -> Product10/1
  Product9/1 -> Product11/3
  Product11/1 -> Subtract3/2
  Subtract3/1 -> Divide2/2
  Add1/1 -> Divide2/1
  Product10/1 -> Add1/2
  Product8/1 -> Product10/3
  Trigonometric Function3/1 -> Product9/1, Product9/3, Product9/2
  Trigonometric Function2/1 -> Product8/1, Product8/3, Product8/2
  Divide2/1 -> Trigonometric Function1/1
  Divide1/1 -> Trigonometric Function/1
  Product7/1 -> Divide1/2
  Product6/1 -> Divide1/1
  Subtract2/1 -> Divide/1
  Product5/1 -> Divide/2, Subtract2/2
  Product4/1 -> Subtract2/1
  Gain/1 -> Subtract1/1
  Product3/1 -> Subtract1/2
  Sqrt/1 -> [P]
  Add/1 -> Sqrt/1
  Product2/1 -> Add/2
  Product1/1 -> Add/1
  Product/1 -> [b]
  Subtract/1 -> Product/2
  Constant/1 -> Subtract/1
  Trigonometric Function1/1 -> lat/1  "lat"
  [a] -> Product11/2
  Subtract1/1 -> Product11/1
  [P] -> Subtract3/1
  [b] -> Product10/2
  [z] -> Add1/1
  [b] -> Product7/2
  [P] -> Product7/1
  Trigonometric Function/1 -> Trigonometric Function2/1, Trigonometric Function3/1
  [a] -> Product6/2
  [z] -> Product6/1
  [f] -> Gain/1, Product3/1, Product3/2
  [b] -> Product5/1, Product5/2
  [a] -> Product4/1, Product4/2
  Demux1/2 -> Product2/1, Product2/2
  Demux1/1 -> Product1/1, Product1/2
  [f] -> Subtract/2
  [a] -> Product/1
  Demux1/3 -> [z]
  pBEE/1 -> Demux1/1
  c_rsma/1 -> [a]
  c_flat/1 -> [f]

== system PILnewH2019/Non-linear Flight Dynamic Model/GRM_Airframe/motion_kinematics/calc_motion_kinematics/calc_transformation_matrix/q31_from_q32_mul_q1/normalize_quaternion ==
  note: Outputs [size]:
      |
      | q_norm [4]
  note: Inputs [size]:
      |
      | q [4]
  q : Inport
  Add : Sum  Inputs=++++
  Demux : Demux  Outputs=[1;1;1;1]
  Math Function : Math  Operator=sqrt  SignedPower=on  SaturateOnIntegerOverflow=on
  Product : Product  Inputs=*/  InputSameDT=on  RndMeth=Zero  SaturateOnIntegerOverflow=on  OutDataTypeStr=Inherit: Same as first input
  Product{1..4} (4 alike) : Product  RndMeth=Zero
  q_normalized : Outport  VectorParamsAs1DForOutWhenUnconnected=off
  wires:
  Math Function/1 -> Product/2
  Add/1 -> Math Function/1
  Product1/1 -> Add/1
  Product2/1 -> Add/2
  Product3/1 -> Add/3
  Product4/1 -> Add/4
  Demux/4 -> Product4/2, Product4/1
  Demux/3 -> Product3/2, Product3/1
  Demux/2 -> Product2/2, Product2/1
  Demux/1 -> Product1/2, Product1/1
  q/1 -> Demux/1, Product/1
  Product/1 -> q_normalized/1

== system PILnewH2019/Non-linear Flight Dynamic Model/GRM_Airframe/motion_kinematics/calc_motion_kinematics/calc_transformation_matrix/q31_from_q32_mul_q2/normalize_quaternion ==
  note: Outputs [size]:
      |
      | q_norm [4]
  note: Inputs [size]:
      |
      | q [4]
  q : Inport
  Add : Sum  Inputs=++++
  Demux : Demux  Outputs=[1;1;1;1]
  Math Function : Math  Operator=sqrt  SignedPower=on  SaturateOnIntegerOverflow=on
  Product : Product  Inputs=*/  InputSameDT=on  RndMeth=Zero  SaturateOnIntegerOverflow=on  OutDataTypeStr=Inherit: Same as first input
  Product{1..4} (4 alike) : Product  RndMeth=Zero
  q_normalized : Outport  VectorParamsAs1DForOutWhenUnconnected=off
  wires:
  Math Function/1 -> Product/2
  Add/1 -> Math Function/1
  Product1/1 -> Add/1
  Product2/1 -> Add/2
  Product3/1 -> Add/3
  Product4/1 -> Add/4
  Demux/4 -> Product4/2, Product4/1
  Demux/3 -> Product3/2, Product3/1
  Demux/2 -> Product2/2, Product2/1
  Demux/1 -> Product1/2, Product1/1
  q/1 -> Demux/1, Product/1
  Product/1 -> q_normalized/1

== system PILnewH2019/Non-linear Flight Dynamic Model/GRM_Airframe/motion_kinematics/calc_motion_kinematics/calc_transformation_matrix/q31_from_q32_mul_q21/normalize_quaternion ==
  note: Outputs [size]:
      |
      | q_norm [4]
  note: Inputs [size]:
      |
      | q [4]
  q : Inport
  Add : Sum  Inputs=++++
  Demux : Demux  Outputs=[1;1;1;1]
  Math Function : Math  Operator=sqrt  SignedPower=on  SaturateOnIntegerOverflow=on
  Product : Product  Inputs=*/  InputSameDT=on  RndMeth=Zero  SaturateOnIntegerOverflow=on  OutDataTypeStr=Inherit: Same as first input
  Product{1..4} (4 alike) : Product  RndMeth=Zero
  q_normalized : Outport  VectorParamsAs1DForOutWhenUnconnected=off
  wires:
  Math Function/1 -> Product/2
  Add/1 -> Math Function/1
  Product1/1 -> Add/1
  Product2/1 -> Add/2
  Product3/1 -> Add/3
  Product4/1 -> Add/4
  Demux/4 -> Product4/2, Product4/1
  Demux/3 -> Product3/2, Product3/1
  Demux/2 -> Product2/2, Product2/1
  Demux/1 -> Product1/2, Product1/1
  q/1 -> Demux/1, Product/1
  Product/1 -> q_normalized/1

== system PILnewH2019/Non-linear Flight Dynamic Model/GRM_Airframe/motion_kinematics/calc_motion_kinematics/earth_rotation/quaternion_integration/Subsystem1 ==
  wEIE : Inport
  qIE : Inport  Port=2
  Add : Sum  Inputs=4
  Constant8 : Constant  Value=0
  Demux : Demux
  Demux1 : Demux  Outputs=3
  Gain : Gain  Gain=0.5
  Product{1..4} (4 alike) : Product
  Product5 : Product  Multiplication=Matrix(*)
  Q_1 : Constant  Value=[0 0 0 1; 0 0 1 0; 0 -1 0 0; -1 0 0 0]
  Q_2 : Constant  Value=[0 0 -1 0; 0 0 0 1; 1 0 0 0; 0 -1 0 0]
  Q_3 : Constant  Value=[0 1 0 0; -1 0 0 0; 0 0 0 1; 0 0 -1 0]
  Q_4 : Constant  Value=[1 0 0 0; 0 1 0 0; 0 0 1 0; 0 0 0 1]
  Vector Concatenate : Concatenate  NumInputs=4
  conjugate_quaternion1 : Subsystem
      mask help: conjugate a quaternion
      mask Help:
      | Name:
      | 
      |     conjugate_quaternion
      | 
      | Description:
      | 
      |     computes the conjugate quaternion
      | 
      | Inputs  [size] [data type] [unit]:
      | 
      |     quaternion q_2_1  [4] [double] [-]
      | 
      | Outputs  [size] [data type] [unit]:
      | 
      |     conjugated quaternion q_1_2  [4] [double] [-]
      mask Display: disp (' conj(q)')
  conjugate_quaternion2 : Subsystem
      mask help: conjugate a quaternion
      mask Help:
      | Name:
      | 
      |     conjugate_quaternion
      | 
      | Description:
      | 
      |     computes the conjugate quaternion
      | 
      | Inputs  [size] [data type] [unit]:
      | 
      |     quaternion q_2_1  [4] [double] [-]
      | 
      | Outputs  [size] [data type] [unit]:
      | 
      |     conjugated quaternion q_1_2  [4] [double] [-]
      mask Display: disp (' conj(q)')
  d_qIE : Outport  VectorParamsAs1DForOutWhenUnconnected=off
  wires:
  qIE/1 -> conjugate_quaternion1/1(q)
  Demux1/3 -> Vector Concatenate/3
  Product2/1 -> Add/2
  Add/1 -> Product5/1
  Demux/4 -> Product4/2  "w4"
  Product4/1 -> Add/4
  Product3/1 -> Add/3
  Q_3/1 -> Product3/1
  Q_1/1 -> Product1/1
  Constant8/1 -> Vector Concatenate/4
  Demux1/1 -> Vector Concatenate/1
  Demux/1 -> Product1/2  "w1"
  Vector Concatenate/1 -> Demux/1
  Q_2/1 -> Product2/1
  Product5/1 -> Gain/1
  Gain/1 -> conjugate_quaternion2/1(q)  "d_qEI"
  Product1/1 -> Add/1
  Q_4/1 -> Product4/1
  Demux/3 -> Product3/2  "w3"
  Demux1/2 -> Vector Concatenate/2
  conjugate_quaternion1/1(q_conj) -> Product5/2  "qEI"
  Demux/2 -> Product2/2  "w2"
  wEIE/1 -> Demux1/1
  conjugate_quaternion2/1(q_conj) -> d_qIE/1  "d_qIE"

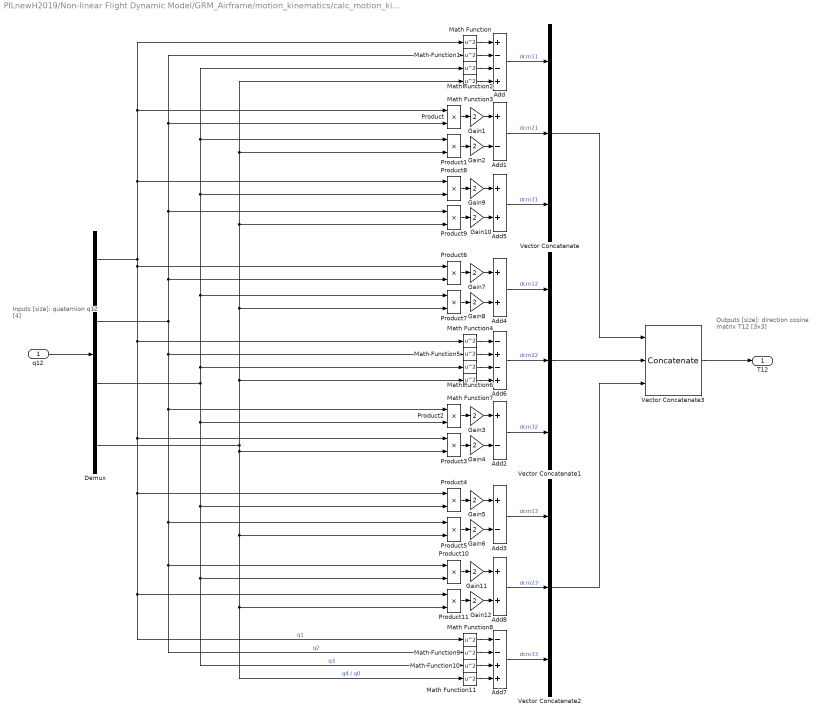
== system PILnewH2019/Non-linear Flight Dynamic Model/GRM_Airframe/motion_kinematics/calc_motion_kinematics/earth_rotation/quaternion_integration/T12_from_q12 ==
  note: Inputs [size]:
      |
      | quaternion q12 [4]
  note: Outputs [size]:
      |
      | direction cosine matrix T12 [3x3]
  q12 : Inport  PortDimensions=4
  Add : Sum  Inputs=+--+
  Add1 : Sum  Inputs=+-
  Add2 : Sum  Inputs=+-
  Add3 : Sum  Inputs=+-
  Add4 : Sum
  Add5 : Sum
  Add6 : Sum  Inputs=-+-+
  Add7 : Sum  Inputs=--++
  Add8 : Sum
  Demux : Demux
  Gain{1..12} (12 alike) : Gain  Gain=2
  Math Function{,1..11} (12 alike) : Math  Operator=square  SignedPower=on  SaturateOnIntegerOverflow=on
  Product{,1..11} (12 alike) : Product
  Vector Concatenate : Concatenate  NumInputs=3
  Vector Concatenate1 : Concatenate  NumInputs=3
  Vector Concatenate2 : Concatenate  NumInputs=3
  Vector Concatenate3 : Concatenate  NumInputs=3  Mode=Multidimensional array  ConcatenateDimension=2
  T12 : Outport  PortDimensions=[3 3]  VectorParamsAs1DForOutWhenUnconnected=off
  wires:
  Product10/1 -> Gain11/1
  Product11/1 -> Gain12/1
  Gain11/1 -> Add8/1
  Gain12/1 -> Add8/2
  Math Function8/1 -> Add7/1
  Math Function9/1 -> Add7/2
  Math Function11/1 -> Add7/4
  Math Function10/1 -> Add7/3
  Math Function4/1 -> Add6/1
  Math Function5/1 -> Add6/2
  Math Function7/1 -> Add6/4
  Math Function6/1 -> Add6/3
  Product8/1 -> Gain9/1
  Product9/1 -> Gain10/1
  Gain9/1 -> Add5/1
  Gain10/1 -> Add5/2
  Product6/1 -> Gain7/1
  Product7/1 -> Gain8/1
  Gain7/1 -> Add4/1
  Gain8/1 -> Add4/2
  Product4/1 -> Gain5/1
  Product5/1 -> Gain6/1
  Gain5/1 -> Add3/1
  Gain6/1 -> Add3/2
  Product2/1 -> Gain3/1
  Product3/1 -> Gain4/1
  Gain3/1 -> Add2/1
  Gain4/1 -> Add2/2
  Gain2/1 -> Add1/2
  Gain1/1 -> Add1/1
  Product1/1 -> Gain2/1
  Product/1 -> Gain1/1
  Math Function3/1 -> Add/4
  Math Function2/1 -> Add/3
  Math Function1/1 -> Add/2
  Math Function/1 -> Add/1
  Add7/1 -> Vector Concatenate2/3  "dcm33"
  Add8/1 -> Vector Concatenate2/2  "dcm23"
  Add3/1 -> Vector Concatenate2/1  "dcm13"
  Add2/1 -> Vector Concatenate1/3  "dcm32"
  Add6/1 -> Vector Concatenate1/2  "dcm22"
  Add4/1 -> Vector Concatenate1/1  "dcm12"
  Add5/1 -> Vector Concatenate/3  "dcm31"
  Add1/1 -> Vector Concatenate/2  "dcm21"
  Add/1 -> Vector Concatenate/1  "dcm11"
  Vector Concatenate1/1 -> Vector Concatenate3/2
  Vector Concatenate2/1 -> Vector Concatenate3/3
  Vector Concatenate/1 -> Vector Concatenate3/1
  Vector Concatenate3/1 -> T12/1
  Demux/4 -> Product3/2, Product11/2, Math Function11/1, Product5/2, Math Function3/1, Product1/2, Product9/2, Product7/2, Math Function7/1  "q4 / q0"
  Demux/3 -> Math Function2/1, Product1/1, Product8/2, Product7/1, Math Function6/1, Product10/2, Math Function10/1, Product4/2, Product2/2  "q3"
  Demux/2 -> Math Function1/1, Product/2, Product9/1, Product6/2, Math Function5/1, Math Function9/1, Product10/1, Product5/1, Product2/1  "q2"
  Demux/1 -> Product6/1, Math Function4/1, Math Function8/1, Product11/1, Product4/1, Product3/1, Math Function/1, Product/1, Product8/1  "q1"
  q12/1 -> Demux/1

== system PILnewH2019/Non-linear Flight Dynamic Model/GRM_Airframe/motion_kinematics/calc_motion_kinematics/earth_rotation/quaternion_integration1/Subsystem1 ==
  wGEG : Inport
  qEG : Inport  Port=2
  Add : Sum  Inputs=4
  Constant8 : Constant  Value=0
  Demux : Demux
  Demux1 : Demux  Outputs=3
  Gain : Gain  Gain=0.5
  Product{1..4} (4 alike) : Product
  Product5 : Product  Multiplication=Matrix(*)
  Q_1 : Constant  Value=[0 0 0 1; 0 0 1 0; 0 -1 0 0; -1 0 0 0]
  Q_2 : Constant  Value=[0 0 -1 0; 0 0 0 1; 1 0 0 0; 0 -1 0 0]
  Q_3 : Constant  Value=[0 1 0 0; -1 0 0 0; 0 0 0 1; 0 0 -1 0]
  Q_4 : Constant  Value=[1 0 0 0; 0 1 0 0; 0 0 1 0; 0 0 0 1]
  Vector Concatenate : Concatenate  NumInputs=4
  conjugate_quaternion1 : Subsystem
      mask help: conjugate a quaternion
      mask Help:
      | Name:
      | 
      |     conjugate_quaternion
      | 
      | Description:
      | 
      |     computes the conjugate quaternion
      | 
      | Inputs  [size] [data type] [unit]:
      | 
      |     quaternion q_2_1  [4] [double] [-]
      | 
      | Outputs  [size] [data type] [unit]:
      | 
      |     conjugated quaternion q_1_2  [4] [double] [-]
      mask Display: disp (' conj(q)')
  conjugate_quaternion2 : Subsystem
      mask help: conjugate a quaternion
      mask Help:
      | Name:
      | 
      |     conjugate_quaternion
      | 
      | Description:
      | 
      |     computes the conjugate quaternion
      | 
      | Inputs  [size] [data type] [unit]:
      | 
      |     quaternion q_2_1  [4] [double] [-]
      | 
      | Outputs  [size] [data type] [unit]:
      | 
      |     conjugated quaternion q_1_2  [4] [double] [-]
      mask Display: disp (' conj(q)')
  d_qEG : Outport  VectorParamsAs1DForOutWhenUnconnected=off
  wires:
  conjugate_quaternion2/1(q_conj) -> d_qEG/1  "d_qEG"
  wGEG/1 -> Demux1/1
  Demux/2 -> Product2/2  "w2"
  conjugate_quaternion1/1(q_conj) -> Product5/2  "qGE"
  Demux1/2 -> Vector Concatenate/2
  Demux/3 -> Product3/2  "w3"
  Q_4/1 -> Product4/1
  Product1/1 -> Add/1
  Gain/1 -> conjugate_quaternion2/1(q)  "d_qGE"
  Product5/1 -> Gain/1
  Q_2/1 -> Product2/1
  Vector Concatenate/1 -> Demux/1
  Demux/1 -> Product1/2  "w1"
  Demux1/1 -> Vector Concatenate/1
  Constant8/1 -> Vector Concatenate/4
  Q_1/1 -> Product1/1
  Q_3/1 -> Product3/1
  Product3/1 -> Add/3
  Product4/1 -> Add/4
  Demux/4 -> Product4/2  "w4"
  Add/1 -> Product5/1
  Product2/1 -> Add/2
  Demux1/3 -> Vector Concatenate/3
  qEG/1 -> conjugate_quaternion1/1(q)

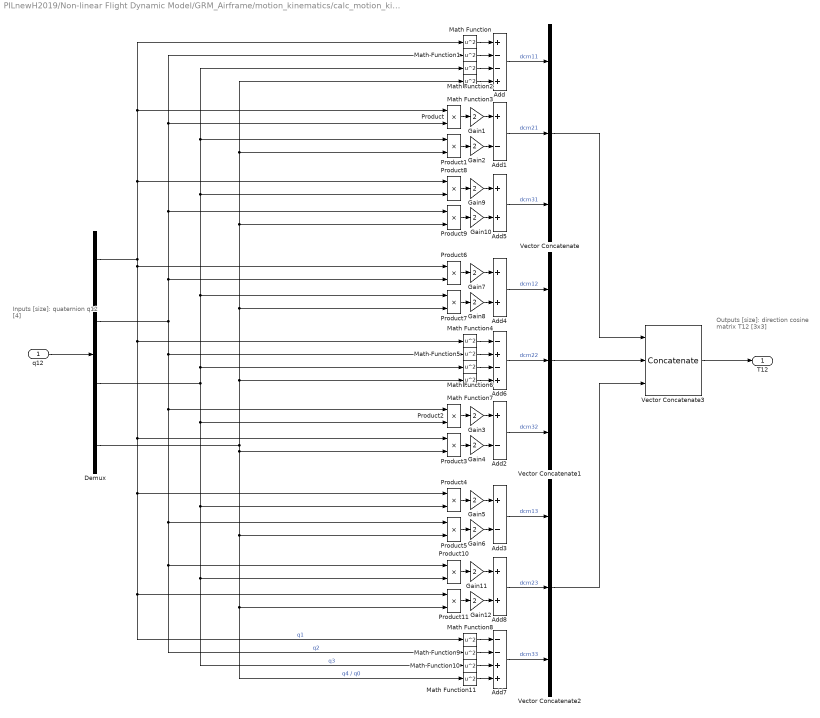
== system PILnewH2019/Non-linear Flight Dynamic Model/GRM_Airframe/motion_kinematics/calc_motion_kinematics/earth_rotation/quaternion_integration1/T12_from_q12 ==
  note: Inputs [size]:
      |
      | quaternion q12 [4]
  note: Outputs [size]:
      |
      | direction cosine matrix T12 [3x3]
  q12 : Inport  PortDimensions=4
  Add : Sum  Inputs=+--+
  Add1 : Sum  Inputs=+-
  Add2 : Sum  Inputs=+-
  Add3 : Sum  Inputs=+-
  Add4 : Sum
  Add5 : Sum
  Add6 : Sum  Inputs=-+-+
  Add7 : Sum  Inputs=--++
  Add8 : Sum
  Demux : Demux
  Gain{1..12} (12 alike) : Gain  Gain=2
  Math Function{,1..11} (12 alike) : Math  Operator=square  SignedPower=on  SaturateOnIntegerOverflow=on
  Product{,1..11} (12 alike) : Product
  Vector Concatenate : Concatenate  NumInputs=3
  Vector Concatenate1 : Concatenate  NumInputs=3
  Vector Concatenate2 : Concatenate  NumInputs=3
  Vector Concatenate3 : Concatenate  NumInputs=3  Mode=Multidimensional array  ConcatenateDimension=2
  T12 : Outport  PortDimensions=[3 3]  VectorParamsAs1DForOutWhenUnconnected=off
  wires:
  Product10/1 -> Gain11/1
  Product11/1 -> Gain12/1
  Gain11/1 -> Add8/1
  Gain12/1 -> Add8/2
  Math Function8/1 -> Add7/1
  Math Function9/1 -> Add7/2
  Math Function11/1 -> Add7/4
  Math Function10/1 -> Add7/3
  Math Function4/1 -> Add6/1
  Math Function5/1 -> Add6/2
  Math Function7/1 -> Add6/4
  Math Function6/1 -> Add6/3
  Product8/1 -> Gain9/1
  Product9/1 -> Gain10/1
  Gain9/1 -> Add5/1
  Gain10/1 -> Add5/2
  Product6/1 -> Gain7/1
  Product7/1 -> Gain8/1
  Gain7/1 -> Add4/1
  Gain8/1 -> Add4/2
  Product4/1 -> Gain5/1
  Product5/1 -> Gain6/1
  Gain5/1 -> Add3/1
  Gain6/1 -> Add3/2
  Product2/1 -> Gain3/1
  Product3/1 -> Gain4/1
  Gain3/1 -> Add2/1
  Gain4/1 -> Add2/2
  Gain2/1 -> Add1/2
  Gain1/1 -> Add1/1
  Product1/1 -> Gain2/1
  Product/1 -> Gain1/1
  Math Function3/1 -> Add/4
  Math Function2/1 -> Add/3
  Math Function1/1 -> Add/2
  Math Function/1 -> Add/1
  Add7/1 -> Vector Concatenate2/3  "dcm33"
  Add8/1 -> Vector Concatenate2/2  "dcm23"
  Add3/1 -> Vector Concatenate2/1  "dcm13"
  Add2/1 -> Vector Concatenate1/3  "dcm32"
  Add6/1 -> Vector Concatenate1/2  "dcm22"
  Add4/1 -> Vector Concatenate1/1  "dcm12"
  Add5/1 -> Vector Concatenate/3  "dcm31"
  Add1/1 -> Vector Concatenate/2  "dcm21"
  Add/1 -> Vector Concatenate/1  "dcm11"
  Vector Concatenate1/1 -> Vector Concatenate3/2
  Vector Concatenate2/1 -> Vector Concatenate3/3
  Vector Concatenate/1 -> Vector Concatenate3/1
  Vector Concatenate3/1 -> T12/1
  Demux/4 -> Product3/2, Product11/2, Math Function11/1, Product5/2, Math Function3/1, Product1/2, Product9/2, Product7/2, Math Function7/1  "q4 / q0"
  Demux/3 -> Math Function2/1, Product1/1, Product8/2, Product7/1, Math Function6/1, Product10/2, Math Function10/1, Product4/2, Product2/2  "q3"
  Demux/2 -> Math Function1/1, Product/2, Product9/1, Product6/2, Math Function5/1, Math Function9/1, Product10/1, Product5/1, Product2/1  "q2"
  Demux/1 -> Product6/1, Math Function4/1, Math Function8/1, Product11/1, Product4/1, Product3/1, Math Function/1, Product/1, Product8/1  "q1"
  q12/1 -> Demux/1

== system PILnewH2019/Non-linear Flight Dynamic Model/GRM_Airframe/rb_eom/calc_bus_flight_dyn_bus_entries/Subsystem2/trafo_E_to_geodetic/Geodetic_altitude ==
  pBEE : Inport
  c_rsma : Inport  Port=2
  c_flat : Inport  Port=3
  lat : Inport  Port=4
  Add : Sum
  Constant : Constant
  Gain : Gain  Gain=2
  Product : Product  Inputs=*/  InputSameDT=on  RndMeth=Zero  SaturateOnIntegerOverflow=on  OutDataTypeStr=Inherit: Same as first input
  Product1 : Product
  Product2 : Product
  Product3 : Product
  Product4 : Product  Inputs=*/  InputSameDT=on  RndMeth=Zero  SaturateOnIntegerOverflow=on  OutDataTypeStr=Inherit: Same as first input
  Product5 : Product  Inputs=3
  Selector : Selector  IndexMode=Zero-based  InputPortWidth=3  IndexOptions=Index vector (dialog)  Indices=0  OutputSizes=1
  Selector1 : Selector  IndexMode=Zero-based  InputPortWidth=3  IndexOptions=Index vector (dialog)  Indices=1  OutputSizes=1
  Sqrt : Sqrt  SaturateOnIntegerOverflow=on
  Sqrt1 : Sqrt  SaturateOnIntegerOverflow=on
  Subtract : Sum  Inputs=+-
  Subtract1 : Sum  Inputs=+-
  Sum : Sum  Inputs=+-  InputSameDT=on  SaturateOnIntegerOverflow=on  OutDataTypeStr=Inherit: Same as first input
  Trigonometric Function : Trigonometry
  cos(latGD) : Trigonometry  Operator=cos
  alt : Outport  VectorParamsAs1DForOutWhenUnconnected=off
  wires:
  Product4/1 -> Sum/2
  Trigonometric Function/1 -> Product5/1, Product5/2
  Product5/1 -> Subtract1/2
  Constant/1 -> Subtract1/1
  Subtract1/1 -> Sqrt1/1
  Sqrt1/1 -> Product4/2
  c_flat/1 -> Gain/1, Product3/2, Product3/1
  Gain/1 -> Subtract/1
  Product3/1 -> Subtract/2
  pBEE/1 -> Selector/1, Selector1/1
  Add/1 -> Sqrt/1
  Product2/1 -> Add/2
  Product1/1 -> Add/1
  Selector1/1 -> Product2/1, Product2/2
  Selector/1 -> Product1/1, Product1/2
  Sum/1 -> alt/1  "alt"
  Product/1 -> Sum/1
  Subtract/1 -> Product5/3
  c_rsma/1 -> Product4/1
  cos(latGD)/1 -> Product/2
  Sqrt/1 -> Product/1
  lat/1 -> cos(latGD)/1, Trigonometric Function/1

== system PILnewH2019/Non-linear Flight Dynamic Model/GRM_Airframe/rb_eom/calc_bus_flight_dyn_bus_entries/Subsystem2/trafo_E_to_geodetic/Geodetic_latitude ==
  pBEE : Inport
  c_rsma : Inport  Port=2
  c_flat : Inport  Port=3
  Add : Sum
  Add1 : Sum
  Constant : Constant
  Demux1 : Demux  Outputs=[1;1;1]
      settings: DisplayOption=none
  Divide : Product  Inputs=*/
  Divide1 : Product  Inputs=*/
  Divide2 : Product  Inputs=*/
  Gain : Gain  Gain=2
  Product{,1..7} (8 alike) : Product
  Product{8..11} (4 alike) : Product  Inputs=3
  Sqrt : Sqrt  SaturateOnIntegerOverflow=on
  Subtract{,1..3} (4 alike) : Sum  Inputs=+-
  Trigonometric Function : Trigonometry  Operator=atan
  Trigonometric Function1 : Trigonometry  Operator=atan
  Trigonometric Function2 : Trigonometry
  Trigonometric Function3 : Trigonometry  Operator=cos
  lat : Outport  VectorParamsAs1DForOutWhenUnconnected=off
  wires:
  Divide/1 -> Product10/1
  Product9/1 -> Product11/3
  Product11/1 -> Subtract3/2
  Subtract3/1 -> Divide2/2
  Add1/1 -> Divide2/1
  Product10/1 -> Add1/2
  Product8/1 -> Product10/3
  Trigonometric Function3/1 -> Product9/1, Product9/3, Product9/2
  Trigonometric Function2/1 -> Product8/1, Product8/3, Product8/2
  Divide2/1 -> Trigonometric Function1/1
  Divide1/1 -> Trigonometric Function/1
  Product7/1 -> Divide1/2
  Product6/1 -> Divide1/1
  Subtract2/1 -> Divide/1
  Product5/1 -> Divide/2, Subtract2/2
  Product4/1 -> Subtract2/1
  Gain/1 -> Subtract1/1
  Product3/1 -> Subtract1/2
  Sqrt/1 -> [P]
  Add/1 -> Sqrt/1
  Product2/1 -> Add/2
  Product1/1 -> Add/1
  Product/1 -> [b]
  Subtract/1 -> Product/2
  Constant/1 -> Subtract/1
  Trigonometric Function1/1 -> lat/1  "lat"
  [a] -> Product11/2
  Subtract1/1 -> Product11/1
  [P] -> Subtract3/1
  [b] -> Product10/2
  [z] -> Add1/1
  [b] -> Product7/2
  [P] -> Product7/1
  Trigonometric Function/1 -> Trigonometric Function2/1, Trigonometric Function3/1
  [a] -> Product6/2
  [z] -> Product6/1
  [f] -> Gain/1, Product3/1, Product3/2
  [b] -> Product5/1, Product5/2
  [a] -> Product4/1, Product4/2
  Demux1/2 -> Product2/1, Product2/2
  Demux1/1 -> Product1/1, Product1/2
  [f] -> Subtract/2
  [a] -> Product/1
  Demux1/3 -> [z]
  pBEE/1 -> Demux1/1
  c_rsma/1 -> [a]
  c_flat/1 -> [f]

== system PILnewH2019/Non-linear Flight Dynamic Model/GRM_Airframe/rb_eom/eom_6dof/Rigid_Body_EOM_6_DOF/Integration/normalize_quaternion ==
  note: Outputs [size]:
      |
      | q_norm [4]
  note: Inputs [size]:
      |
      | q [4]
  q : Inport
  Add : Sum  Inputs=++++
  Demux : Demux  Outputs=[1;1;1;1]
  Math Function : Math  Operator=sqrt  SignedPower=on  SaturateOnIntegerOverflow=on
  Product : Product  Inputs=*/  InputSameDT=on  RndMeth=Zero  SaturateOnIntegerOverflow=on  OutDataTypeStr=Inherit: Same as first input
  Product{1..4} (4 alike) : Product  RndMeth=Zero
  q_normalized : Outport  VectorParamsAs1DForOutWhenUnconnected=off
  wires:
  Math Function/1 -> Product/2
  Add/1 -> Math Function/1
  Product1/1 -> Add/1
  Product2/1 -> Add/2
  Product3/1 -> Add/3
  Product4/1 -> Add/4
  Demux/4 -> Product4/2, Product4/1
  Demux/3 -> Product3/2, Product3/1
  Demux/2 -> Product2/2, Product2/1
  Demux/1 -> Product1/2, Product1/1
  q/1 -> Demux/1, Product/1
  Product/1 -> q_normalized/1
